simulink model "ElectricPowertrain_SLX"  (R2017b)
settings: Solver=VariableStepAuto  StartTime=0.0  StopTime=10.0  RelTol=1e-3
undefined symbols (not defined in the file): b_mc, J_mc, K_c, P_2_0, r_1, r_2, T_m_0, Ts, W_w_0, x_5_0
settings Model: Creator=Luca  LastModifiedBy=Luca

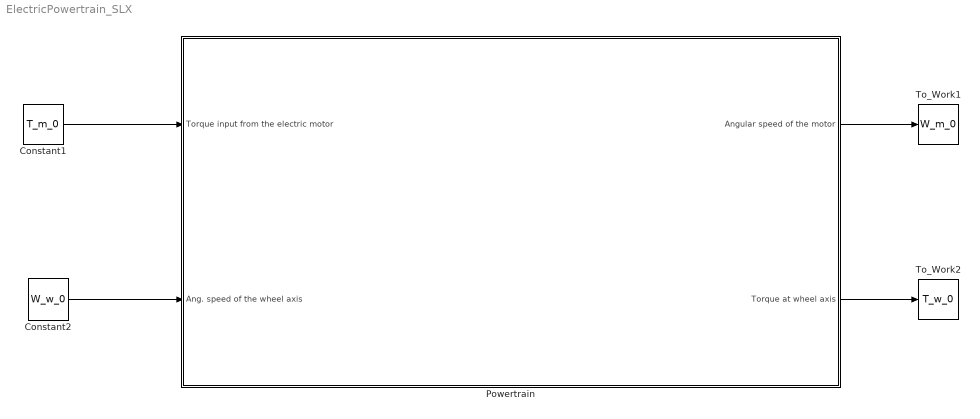
== system ElectricPowertrain_SLX ==
  Constant1 : Constant  Value=T_m_0
  Constant2 : Constant  Value=W_w_0
  Powertrain : Subsystem
  To_Work1 : ToWorkspace  VariableName=W_m_0  SampleTime=Ts
      settings: MaxDataPoints=10000
  To_Work2 : ToWorkspace  VariableName=T_w_0  SampleTime=Ts
      settings: MaxDataPoints=10000
  wires:
  Constant1/1 -> Powertrain/1(Torque input from the electric motor)
  Powertrain/1(Angular speed of the motor) -> To_Work1/1
  Powertrain/2(Torque at wheel axis) -> To_Work2/1
  Constant2/1 -> Powertrain/2(Ang. speed of the wheel axis)

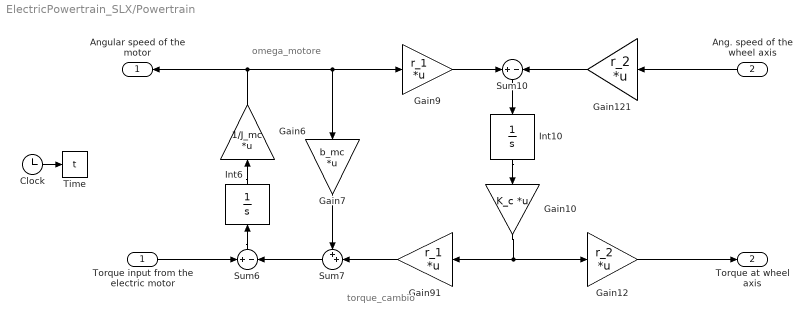
== system ElectricPowertrain_SLX/Powertrain ==
  note: omega_motore
  note: torque_cambio
  Torque input from the electric motor : Inport
  Ang. speed of the wheel axis : Inport  Port=2
  Clock : Clock
  Gain10 : Gain  Gain=K_c  Multiplication=Matrix(K*u)  SaturateOnIntegerOverflow=on  OutDataTypeStr=Inherit: Same as input  ParamDataTypeStr=Inherit: Same as input
  Gain12 : Gain  Gain=r_2  Multiplication=Matrix(K*u)  SaturateOnIntegerOverflow=on  OutDataTypeStr=Inherit: Same as input  ParamDataTypeStr=Inherit: Same as input
  Gain121 : Gain  Gain=r_2  Multiplication=Matrix(K*u)  SaturateOnIntegerOverflow=on  OutDataTypeStr=Inherit: Same as input  ParamDataTypeStr=Inherit: Same as input
  Gain6 : Gain  Gain=1/J_mc  Multiplication=Matrix(K*u)  SaturateOnIntegerOverflow=on  OutDataTypeStr=Inherit: Same as input  ParamDataTypeStr=Inherit: Same as input
  Gain7 : Gain  Gain=b_mc  Multiplication=Matrix(K*u)  SaturateOnIntegerOverflow=on  OutDataTypeStr=Inherit: Same as input  ParamDataTypeStr=Inherit: Same as input
  Gain9 : Gain  Gain=r_1  Multiplication=Matrix(K*u)  SaturateOnIntegerOverflow=on  OutDataTypeStr=Inherit: Same as input  ParamDataTypeStr=Inherit: Same as input
  Gain91 : Gain  Gain=r_1  Multiplication=Matrix(K*u)  SaturateOnIntegerOverflow=on  OutDataTypeStr=Inherit: Same as input  ParamDataTypeStr=Inherit: Same as input
  Int10 : Integrator  InitialCondition=x_5_0
  Int6 : Integrator  InitialCondition=P_2_0
  Sum10 : Sum  Inputs=+|-  SaturateOnIntegerOverflow=on  InputSameDT=on  OutDataTypeStr=Inherit: Same as first input
  Sum6 : Sum  Inputs=+|-  SaturateOnIntegerOverflow=on  InputSameDT=on  OutDataTypeStr=Inherit: Same as first input
  Sum7 : Sum  Inputs=++|  SaturateOnIntegerOverflow=on  InputSameDT=on  OutDataTypeStr=Inherit: Same as first input
  Time : ToWorkspace  VariableName=t  SampleTime=Ts
      settings: MaxDataPoints=10000
  Angular speed of the motor : Outport
  Torque at wheel axis : Outport  Port=2
  wires:
  Clock/1 -> Time/1
  Torque input from the electric motor/1 -> Sum6/1
  Sum7/1 -> Sum6/2
  Sum6/1 -> Int6/1
  Int6/1 -> Gain6/1
  Gain7/1 -> Sum7/1
  Gain91/1 -> Sum7/2
  Gain6/1 -> Angular speed of the motor/1, Gain7/1, Gain9/1
  Gain121/1 -> Sum10/2
  Gain9/1 -> Sum10/1
  Int10/1 -> Gain10/1
  Sum10/1 -> Int10/1
  Gain10/1 -> Gain12/1, Gain91/1
  Gain12/1 -> Torque at wheel axis/1
  Ang. speed of the wheel axis/1 -> Gain121/1
